simulink model "simulation"  (R2023a)
settings: Solver=VariableStepAuto  StartTime=0.0  StopTime=10.0  RelTol=1e-3
settings Model: Creator=poudell  LastModifiedBy=poudell

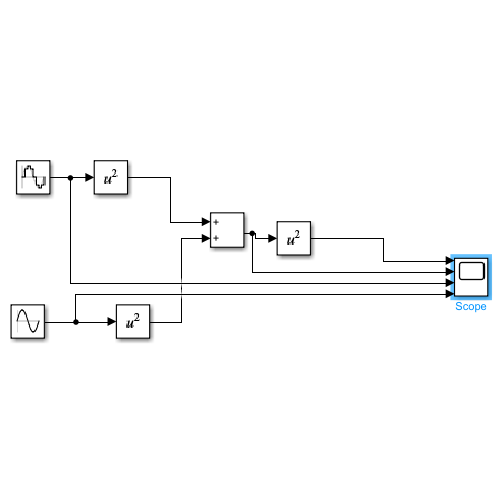
[thumbnail: Simulink's stored preview of the top-level diagram]
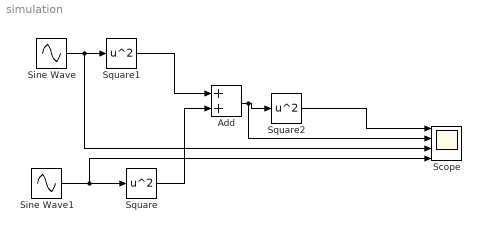
== system simulation ==
  Add : Sum
  Scope : Scope  NumInputPorts=4
  Sine Wave : Sin  Frequency=2*pi*20  SampleTime=1/200
  Sine Wave1 : Sin  Frequency=2*pi*30  SampleTime=0
  Square : Math  Operator=square
  Square1 : Math  Operator=square
  Square2 : Math  Operator=square
  wires:
  Sine Wave1/1 -> Scope/4, Square/1
  Sine Wave/1 -> Scope/3, Square1/1
  Square1/1 -> Add/1
  Square/1 -> Add/2
  Add/1 -> Scope/2, Square2/1
  Square2/1 -> Scope/1
